simulink model "cardetect"  (Simulink 7.9)
settings: Solver=ode45  StartTime=0.0  StopTime=10.0  RelTol=1e-3
values from neighbouring files (symbols this model uses):
  magnitude = flow .* conj(flow)    [opticalflow.m]
undefined symbols (not defined in the file or in its folder): Horn, Rec, Schunck, SDTV, strel
libraries: visionsinks x4, visiontextngfix x3, visionstatistics x3, visionanalysis x2, visionmorphops x2, visionconversions x1, dspvision x1
settings Model: Creator=Dynamic  LastModifiedBy=Dynamic

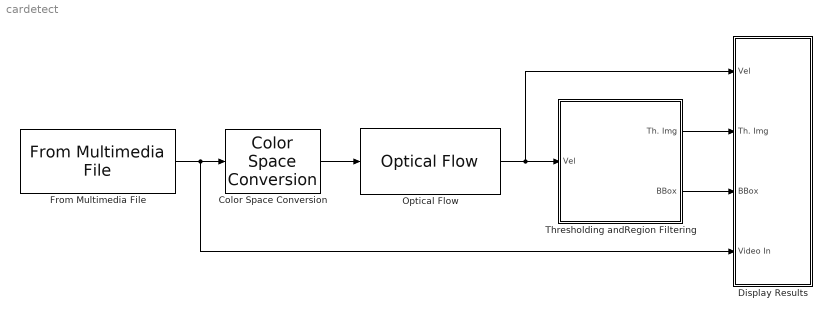
== system cardetect ==
  Color Space Conversion : visionconversions/Color Space  Conversion  conversion=Obsolete  conversionActive=R'G'B' to intensity  wp_str=D65  rec=Rec. 601 (SDTV)  sys=1125/60/2:1  imagePorts=One multidimensional signal
  Display Results : Subsystem
  From Multimedia File : dspvision/From Multimedia File  inputFilename=viptraffic.avi  loop=on  numPlays=inf  outputStreams=Video only  videoDataType=single  audioDataType=int16  inheritSampleTime=on  userDefinedSampleTime=1/40  noAudioOutput=off  isIntensityVideo=off  fourcc=RGB  colorVideoFormat=One multidimensional signal  outputEOF=off  dataOrg=Column-major  audioFrameSize=1024  computeAudioFrameSize=off  outSamplingMode=Frame based
  Optical Flow : visionanalysis/Optical Flow  method=Horn-Schunck  gradMethod=Difference filter [-1 1]  which2img=Current frame and N-th frame back  N=1  outVelForm=Horizontal and vertical components in complex form  lambda=1  stop_criteria=When maximum number of iterations is reached  maxAllowAbsDiff=eps  maxIter=10  numInports=3  sigmaS=1.5  sigmaW=1  eigTh=0.0039  discardNormalFlow=off  outputCurrentImage=off  prodOutputMode=Binary point scaling  prodOutputWordLength=32  prodOutputFracLength=20  outputMode=Binary point scaling  outputWordLength=32  outputFracLength=20  roundingMode=Nearest  overflowMode=on
  Thresholding andRegion Filtering : Subsystem
  wires:
  Optical Flow/1 -> Display Results/1(Vel), Thresholding andRegion Filtering/1(Vel)
  Color Space Conversion/1 -> Optical Flow/1
  From Multimedia File/1 -> Color Space Conversion/1, Display Results/4(Video In)
  Thresholding andRegion Filtering/1(Th. Img) -> Display Results/2(Th. Img)
  Thresholding andRegion Filtering/2(BBox) -> Display Results/3(BBox)

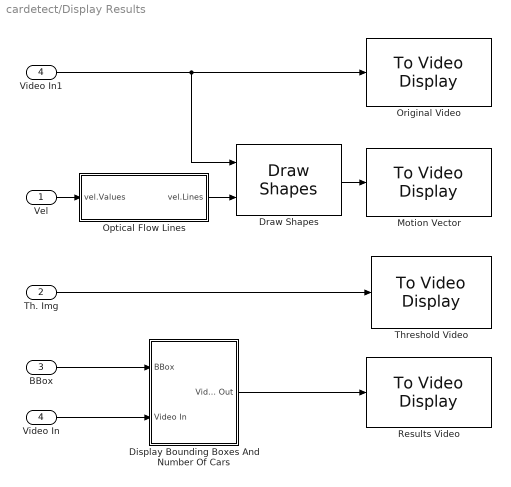
== system cardetect/Display Results ==
  Vel : Inport
  Th. Img : Inport  Port=2
  BBox : Inport  Port=3
  Video In : Inport  Port=4
  Display Bounding Boxes And Number Of Cars : Subsystem
  Draw Shapes : visiontextngfix/Draw Shapes  shape=Lines  fill=off  fillClrSource=Specify via dialog  display=User-specified value  intensity=200  color=[255 255 0]  opacity=0.6  viewport=Entire image  antialiasing=off  inType=Obsolete  imagePorts=One multidimensional signal  prodOutputMode=Binary point scaling  prodOutputWordLength=32  prodOutputFracLength=14  memoryMode=Specify word length  memoryWordLength=16  memoryFracLength=15  roundingMode=Floor  overflowMode=off
  Motion Vector : visionsinks/To Video Display  inputType=Obsolete  imagePorts=One multidimensional signal  OutputDevice=On-screen video monitor  fullScreen=off  videoWindowX=345  videoWindowY=152  saveWindowSize=off  videoWindowWidth=168  videoWindowHeight=147  dataOrg=Column-major  openAtMdlStart=on  isWindowOpen=off  inputColorFormat=RGB
  Optical Flow Lines : Subsystem  mask(Optical Flow Lines){scaleFactor=20}
      mask prompts: scaleFactor "Motion vector gain:"
      mask help: Generates the coordinate points of optical flow lines.
      mask Help: Generates the coordinate points of optical flow lines. Look under its mask to see the implementation details.
  Original Video : visionsinks/To Video Display  inputType=Obsolete  imagePorts=One multidimensional signal  OutputDevice=On-screen video monitor  fullScreen=off  videoWindowX=178  videoWindowY=151  saveWindowSize=off  videoWindowWidth=168  videoWindowHeight=147  dataOrg=Column-major  openAtMdlStart=on  isWindowOpen=off  inputColorFormat=RGB
  Results Video : visionsinks/To Video Display  inputType=Obsolete  imagePorts=One multidimensional signal  OutputDevice=On-screen video monitor  fullScreen=off  videoWindowX=680  videoWindowY=154  saveWindowSize=off  videoWindowWidth=168  videoWindowHeight=147  dataOrg=Column-major  openAtMdlStart=on  isWindowOpen=off  inputColorFormat=RGB
  Threshold Video : visionsinks/To Video Display  inputType=Intensity  imagePorts=One multidimensional signal  OutputDevice=On-screen video monitor  fullScreen=off  videoWindowX=513  videoWindowY=152  saveWindowSize=off  videoWindowWidth=168  videoWindowHeight=147  dataOrg=Column-major  openAtMdlStart=on  isWindowOpen=off  inputColorFormat=RGB
  Video In1 : InportShadow  Port=4
  wires:
  Video In/1 -> Display Bounding Boxes And Number Of Cars/2(Video In)
  Th. Img/1 -> Threshold Video/1
  BBox/1 -> Display Bounding Boxes And Number Of Cars/1(BBox)
  Display Bounding Boxes And Number Of Cars/1(Video Out) -> Results Video/1
  Optical Flow Lines/1(vel.Lines) -> Draw Shapes/2
  Vel/1 -> Optical Flow Lines/1(vel.Values)
  Draw Shapes/1 -> Motion Vector/1
  Video In1/1 -> Original Video/1, Draw Shapes/1

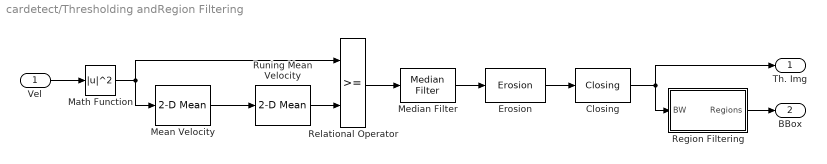
== system cardetect/Thresholding andRegion Filtering ==
  Vel : Inport
  Closing : visionmorphops/Closing  nhoodsrc=Specify via dialog  strel=strel('line',6,45)
  Erosion : visionmorphops/Erosion  nhoodsrc=Specify via dialog  strel=strel('square',4)
  Math Function : Math  Operator=magnitude^2  SaturateOnIntegerOverflow=on
  Mean Velocity : visionstatistics/2-D Mean  run=off  reset_popup=None  directionMode=Entire input  dimension=1  treatSBRowAsCol=on  roiEnable=off  roiType=Rectangles  roiPortion=Entire ROI  roiOutput=Individual statistics for each ROI  roiFlag=off  outputDataTypeStr=Inherit: Same as accumulator  outputLastDataTypeStr=Inherit: Same as accumulator  outputMin=[]  outputMax=[]  accumMode=Binary point scaling  accumWordLength=32  accumFracLength=0  accumDataTypeStr=fixdt([],32,0)  accumLastDataTypeStr=fixdt([],32,0)  roundingMode=Floor  overflowMode=off
  Median Filter : visionanalysis/Median Filter  nghbood=[3 3]  outSize=Same as input port I  padType=Constant  padSrc=Specify via dialog  padVal=1  roundingMode=Floor  overflowMode=off
  Region Filtering : Subsystem
  Relational Operator : RelationalOperator  OutDataTypeStr=boolean
  Runing Mean Velocity : visionstatistics/2-D Mean  run=on  reset_popup=None  directionMode=Entire input  dimension=1  treatSBRowAsCol=on  roiEnable=off  roiType=Rectangles  roiPortion=Entire ROI  roiOutput=Individual statistics for each ROI  roiFlag=off  outputDataTypeStr=Inherit: Same as accumulator  outputLastDataTypeStr=Inherit: Same as accumulator  outputMin=[]  outputMax=[]  accumMode=Binary point scaling  accumWordLength=32  accumFracLength=0  accumDataTypeStr=fixdt([],32,0)  accumLastDataTypeStr=fixdt([],32,0)  roundingMode=Floor  overflowMode=off
  Th. Img : Outport
  BBox : Outport  Port=2
  wires:
  Math Function/1 -> Relational Operator/1, Mean Velocity/1
  Relational Operator/1 -> Median Filter/1
  Vel/1 -> Math Function/1
  Region Filtering/1(Regions) -> BBox/1
  Median Filter/1 -> Erosion/1
  Closing/1 -> Region Filtering/1(BW), Th. Img/1
  Mean Velocity/1 -> Runing Mean Velocity/1
  Runing Mean Velocity/1 -> Relational Operator/2
  Erosion/1 -> Closing/1

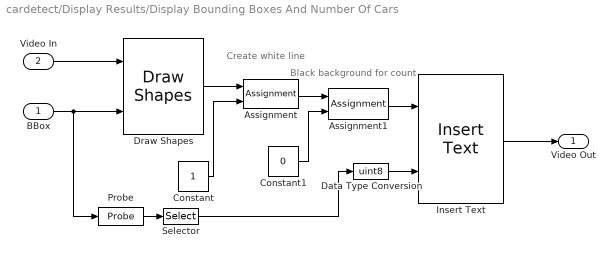
== system cardetect/Display Results/Display Bounding Boxes And Number Of Cars ==
  note: Create white
      | line
  note: Black background
      | for count
  BBox : Inport
  Video In : Inport  Port=2
  Assignment : Assignment  NumberOfDimensions=3  IndexOptions=Index vector (dialog),Assign all,Assign all  Indices=[22:23],[],[]  OutputSizes=1, 1
  Assignment1 : Assignment  NumberOfDimensions=3  IndexOptions=Index vector (dialog),Index vector (dialog),Assign all  Indices=[1:15],[1:30],[]  OutputSizes=1, 1
  Constant : Constant  OutDataTypeStr=single
  Constant1 : Constant  Value=0  OutDataTypeStr=single
  Data Type Conversion : DataTypeConversion  OutDataTypeStr=uint8
  Draw Shapes : visiontextngfix/Draw Shapes  shape=Rectangles  fill=off  fillClrSource=Specify via dialog  display=User-specified value  intensity=200  color=[0 1 0]  opacity=0.6  viewport=Entire image  antialiasing=off  inType=Obsolete  imagePorts=One multidimensional signal  prodOutputMode=Binary point scaling  prodOutputWordLength=32  prodOutputFracLength=14  memoryMode=Specify word length  memoryWordLength=16  memoryFracLength=15  roundingMode=Floor  overflowMode=off
  Insert Text : visiontextngfix/Insert Text  inputType=Obsolete  theText='%4d'  fontFace=LucidaTypewriterRegular  dummyVar1=0  blockFontSize=12  antiAliased=on  getTextLocFrom=Specify via dialog  textLoc=[1 1]  getTextColorFrom=Specify via dialog  textColor=[1 1 1]  getTextIntensityFrom=Specify via dialog  textIntensity=1  getTextOpacityFrom=Specify via dialog  textOpacity=1.0  dummyVar2=0  dummyVar3=0  dummyVar4=0  imagePorts=One multidimensional signal  isInputTransposed=off
  Probe : Probe  ProbeWidth=off  ProbeSampleTime=off  ProbeComplexSignal=off  ProbeSignalDimensions=on  ProbeWidthDataType=uint8
  Selector : Selector  NumberOfDimensions=2  InputPortWidth=3  IndexOptions=Index vector (dialog),Index vector (dialog)  Indices=1,1  OutputSizes=99,1
  Video Out : Outport
  wires:
  Data Type Conversion/1 -> Insert Text/2
  Selector/1 -> Data Type Conversion/1
  Probe/1 -> Selector/1
  Assignment1/1 -> Insert Text/1
  Insert Text/1 -> Video Out/1
  Video In/1 -> Draw Shapes/1
  Constant1/1 -> Assignment1/2
  Constant/1 -> Assignment/2
  Assignment/1 -> Assignment1/1
  Draw Shapes/1 -> Assignment/1
  BBox/1 -> Probe/1, Draw Shapes/2

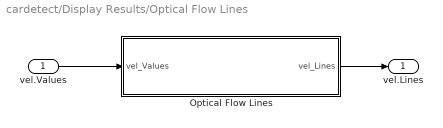
== system cardetect/Display Results/Optical Flow Lines ==
  vel.Values : Inport
  Optical Flow Lines : MATLAB Function  TreatAsAtomicUnit=on
  vel.Lines : Outport
  wires:
  vel.Values/1 -> Optical Flow Lines/1(vel_Values)
  Optical Flow Lines/1(vel_Lines) -> vel.Lines/1

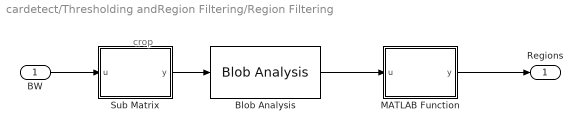
== system cardetect/Thresholding andRegion Filtering/Region Filtering ==
  note: crop
  BW : Inport
  Blob Analysis : visionstatistics/Blob Analysis  Tag=vipblks_row_conv  area=off  centroid=off  bBox=on  majorAxis=off  minorAxis=off  angle=off  eccentricity=off  equivDiameterSq=off  extent=off  perimeter=off  maxBlobs=80  warnIfNumBlobsExceeded=on  isCount=off  useMinArea=on  minArea=300  useMaxArea=on  maxArea=3600  excludeBorderBlob=on  outDT=double  isOutVarDim=on  isFill=on  fillValues=-1  conn=8  isLabel=off  outputMode=Binary point scaling  outputWordLength=32  outputFracLength=16  firstCoeffMode=Binary point scaling  firstCoeffWordLength=16  firstCoeffFracLength=14  secondCoeffMode=Binary point scaling  secondCoeffWordLength=32  secondCoeffFracLength=16  accumMode=Binary point scaling  accumWordLength=32  accumFracLength=0  prodOutputMode=Binary point scaling  prodOutputWordLength=32  prodOutputFracLength=16  roundingMode=Floor  overflowMode=off
  MATLAB Function : MATLAB Function  TreatAsAtomicUnit=on
  Sub Matrix : MATLAB Function  TreatAsAtomicUnit=on
  Regions : Outport
  wires:
  Blob Analysis/1 -> MATLAB Function/1(u)
  BW/1 -> Sub Matrix/1(u)
  MATLAB Function/1(y) -> Regions/1
  Sub Matrix/1(y) -> Blob Analysis/1

== matlab function Display Results/Optical Flow Lines/Optical Flow Lines ==
  data: vel_Values input double; vel_Lines output double; scaleFactor parameter double size=1
function vel_Lines=OpticalFlowLines(vel_Values, scaleFactor) 

% Generates the coordinate points of optical flow lines

persistent first_time;
persistent X;
persistent Y;
persistent RV;
persistent CV;
if isempty(first_time)
    first_time     = 1;
    %% user may change the following three parameters
    borderOffset   = 5;
    decimFactorRow = 5;
    decimFactorCol = 5;    
    %%
    [R C] = size(vel_Values);
    RV = borderOffset:decimFactorRow:(R-borderOffset);   
    CV = borderOffset:decimFactorCol:(C-borderOffset);
    [Y X] = meshgrid(CV,RV);
end

tmp = vel_Values(RV,CV);
tmp = tmp.*scaleFactor;
vel_Lines = [Y(:), X(:), Y(:)+real(tmp(:)), X(:)+imag(tmp(:))];

== matlab function Thresholding andRegion Filtering/Region Filtering/MATLAB Function ==
  data: u input double size=[80 4] [..320]; y output double size=size(u) [..320]; line_row parameter double
function y = fcn(u, line_row)
%#codegen
dim=size(u);
repVector = zeros(dim);
repVector=repmat([0 line_row 0 0],dim(1),1); 

y = int32(u+int32(repVector));

== matlab function Thresholding andRegion Filtering/Region Filtering/Sub Matrix ==
  data: u input double; y output double; line_row parameter double
function y = fcn(u, line_row)
%#codegen

l=size(u);

y = u(line_row:l(1),:);
